simulink model "ABS"  (Simulink 7.4)
settings: Solver=ode45  StartTime=0.0  StopTime=15  RelTol=1e-3
settings Model: Creator=carlj  LastModifiedBy=alesch
settings DataIOCC: LimitDataPoints=off  SaveOutput=off  SaveTime=off
settings OptimizationCC: InlineParams=on  InitFltsAndDblsToZero=on  EfficientMapNaN2IntZero=off
settings DebuggingCC: IntegerOverflowMsg=none  StrictBusMsg=ErrorLevel1
settings HardwareCC: TargetEndianess=LittleEndian  TargetHWDeviceType=MATLAB Host  ProdEqTarget=off
settings RTWCC: SystemTargetFile=modelrefsim.tlc  TemplateMakefile=modelrefsim_default_tmf  RTWVerbose=off  ProcessScript=modelrefsim_make_rtw_hook  IncludeBusHierarchyInRTWFileBlockHierarchyMap=on
settings CodeAppCC: GenerateComments=off  MaxIdLength=128  SimulinkBlockComments=off
settings ERTTargetCC: MultiwordLength=2048  CombineOutputUpdateFcns=off  SupportContinuousTime=on  SupportNonInlinedSFcns=on  InlinedParameterPlacement=NonHierarchical  RTWCAPISignals=on  RTWCAPIStates=on  ConvertIfToSwitch=off

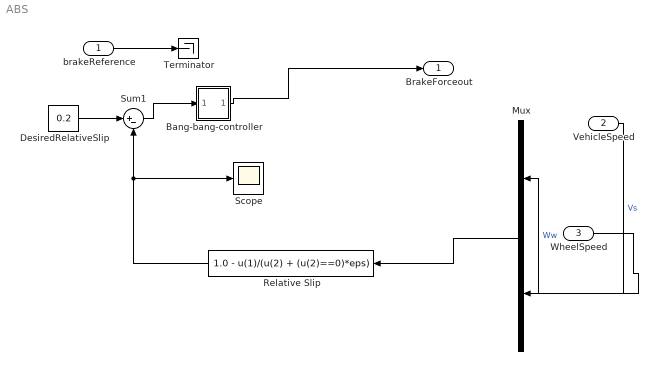
== system ABS ==
  brakeReference : Inport  OutDataType=fixdt(1, 16)  OutScaling=2^0
  VehicleSpeed : Inport  Port=2  PortDimensions=1  SampleTime=0  DataType=double  OutDataTypeStr=double
  WheelSpeed : Inport  Port=3  PortDimensions=1  SampleTime=0  DataType=double  OutDataTypeStr=double
  Bang-bang-controller : Subsystem
      mask Type: Sign
      mask Description: y = sign(x)
      mask Help: Sign Function:\n\t\t\ty = 1 if x > 0\n\t\t\ty = 0 if x = 0\n\t\t\ty = -1 if x < 0
      mask Display: plot(-50,-50,50,50,[-50,50],[0,0],[0,0],[-50,50],[-40,0],[-30,-30],[0,40],[30,30])
  DesiredRelativeSlip : Constant  Value=0.2  OutDataType=sfix(16)  OutScaling=2^0
  Mux : Mux  Inputs=2
  Relative Slip : Fcn  Expr=1.0 - u(1)/(u(2) + (u(2)==0)*eps)
  Scope : Scope
  Sum1 : Sum  Inputs=|+-  OutDataType=sfix(16)  OutScaling=2^0  SaturateOnIntegerOverflow=on  InputSameDT=on  OutDataTypeStr=Inherit: Same as first input
  Terminator : Terminator
  BrakeForceout : Outport  PortDimensions=1  SampleTime=[0,1]  DataType=double  OutDataTypeStr=double
  wires:
  VehicleSpeed/1 -> Mux/2  "Vs"
  WheelSpeed/1 -> Mux/1  "Ww"
  Mux/1 -> Relative Slip/1
  Relative Slip/1 -> Scope/1, Sum1/2
  Bang-bang-controller/1(out_1) -> BrakeForceout/1
  Sum1/1 -> Bang-bang-controller/1(in_1)
  DesiredRelativeSlip/1 -> Sum1/1
  brakeReference/1 -> Terminator/1

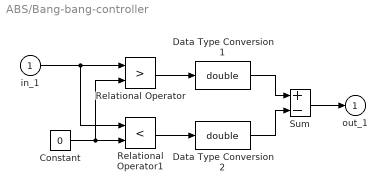
== system ABS/Bang-bang-controller ==
  in_1 : Inport  OutDataType=sfix(16)  OutScaling=2^0
  Constant : Constant  Value=0  OutDataType=sfix(16)  OutScaling=2^0
  Data Type Conversion1 : DataTypeConversion  OutDataTypeMode=double  OutDataType=sfix(16)  OutScaling=2^0  OutDataTypeStr=double  SaturateOnIntegerOverflow=on  RndMeth=Zero
  Data Type Conversion2 : DataTypeConversion  OutDataTypeMode=double  OutDataType=sfix(16)  OutScaling=2^0  OutDataTypeStr=double  SaturateOnIntegerOverflow=on  RndMeth=Zero
  Relational Operator : RelationalOperator  Operator=>  InputSameDT=on
  Relational Operator1 : RelationalOperator  Operator=<  InputSameDT=on
  Sum : Sum  Inputs=+-  OutDataType=sfix(16)  OutScaling=2^0  SaturateOnIntegerOverflow=on  InputSameDT=on  OutDataTypeStr=Inherit: Same as first input
  out_1 : Outport  OutDataType=sfix(16)  OutScaling=2^0  InitialOutput=0
  wires:
  in_1/1 -> Relational Operator/1, Relational Operator1/1
  Constant/1 -> Relational Operator1/2, Relational Operator/2
  Relational Operator1/1 -> Data Type Conversion2/1
  Relational Operator/1 -> Data Type Conversion1/1
  Sum/1 -> out_1/1
  Data Type Conversion1/1 -> Sum/1
  Data Type Conversion2/1 -> Sum/2
